simulink model "sampleModel1432_1_sub_sub"  (R2023a)
settings: Solver=VariableStepAuto  StartTime=0.0  StopTime=10.0  RelTol=1e-3
libraries: hdlsllib x5, simulink x2
settings Model: Creator=user1  LastModifiedBy=user1
settings OptimizationCC: BlockReduction=off  ConditionallyExecuteInputs=off

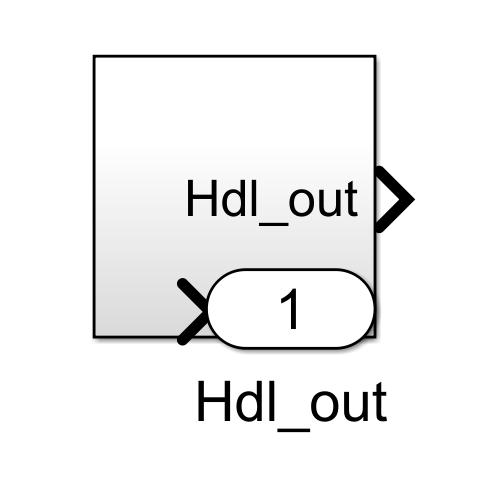
[thumbnail: Simulink's stored preview of the top-level diagram]
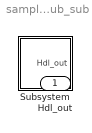
== system sampleModel1432_1_sub_sub ==
  Subsystem : Subsystem
  Hdl_out : Outport  OutDataTypeStr=uint8

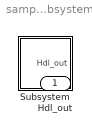
== system sampleModel1432_1_sub_sub/Subsystem ==
  Subsystem : Subsystem
  Hdl_out : Outport  OutDataTypeStr=uint8

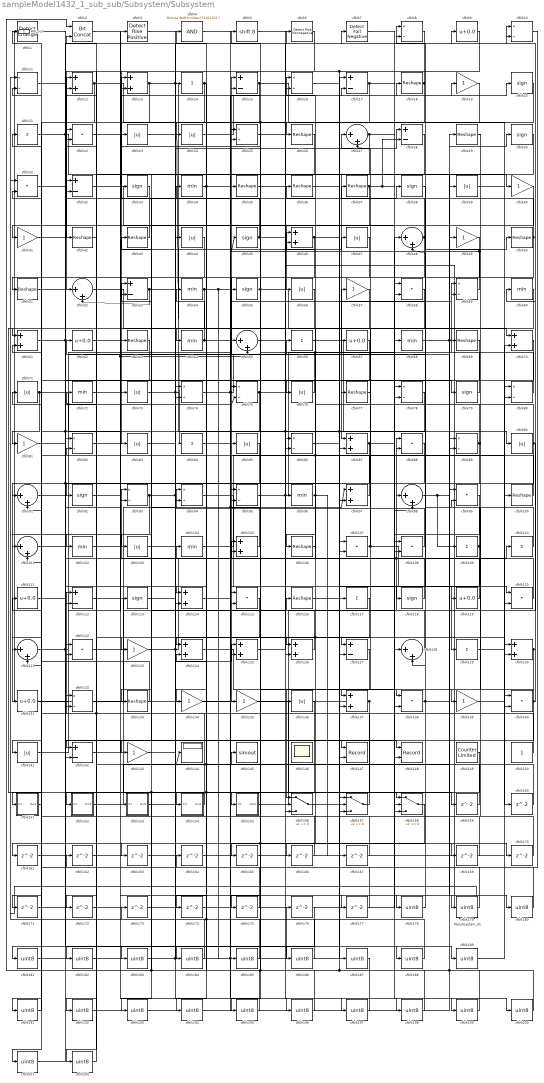
== system sampleModel1432_1_sub_sub/Subsystem/Subsystem ==
  Mysubsystem_31 : Subsystem  TreatAsAtomicUnit=on  RTWFcnName=Mysubsystem_31
      settings: RTWFcnNameOpts=User specified  RTWFileNameOpts=Use function name
  cfblk1 : simulink/Logic and Bit Operations/Detect Change  vinit=0  OutDataTypeStr=uint8
      settings: LibrarySourceBlock=|
      | hdlsllib/Logic and Bit
      | Operations/Detect
      | Change
  cfblk{8,10..11,16,25,59,74..75,78,80,82,86,89,93..95,132} (17 alike) : Product  Inputs=*/  OutDataTypeStr=uint8  RndMeth=Zero  SaturateOnIntegerOverflow=on
  cfblk{18,26,29,35..37,42..43,50..51,63,69,77,100,106,116,133} (17 alike) : Reshape
  cfblk{27,48,52,65,91,98,101,121,128} (9 alike) : Sum  Inputs=|++  OutDataTypeStr=uint8
  cfblk{34,54,60,64,68,72,96,102,104} (9 alike) : MinMax  OutDataTypeStr=uint8
  cfblk{23..24,39,44,47,56,71,73,76,83,85,90,103,136,141} (15 alike) : Abs  OutDataTypeStr=uint8  SaturateOnIntegerOverflow=off
  cfblk{12..13,46,61,70,87,97,105,114,124..126,130,137} (14 alike) : Sum  OutDataTypeStr=uint8
  cfblk{22,31,58,88,99,107..108,115,120,122,138,140} (12 alike) : DotProduct  OutDataTypeStr=uint8
  cfblk{14,21,66,84,109..110,117,129} (8 alike) : Sum  Inputs=+  OutDataTypeStr=uint8
  cfblk{9,62,67,111,119,131} (6 alike) : Bias  Bias=0.0  SaturateOnIntegerOverflow=off
  cfblk{15,17,28,32,53,112,127,142} (8 alike) : Sum  Inputs=+-  OutDataTypeStr=uint8
  cfblk{20,30,33,38,45,55,79,92,113,118} (10 alike) : Signum
  cfblk{19,40..41,49,57,81,123,134..135,139,143} (11 alike) : Gain  OutDataTypeStr=uint8
  cfblk144 : Display
  cfblk145 : ToWorkspace  VariableName=simout  SaveFormat=Timeseries  SampleTime=-1
  cfblk146 : Scope
      settings: Floating=on
  cfblk147 : Record  FileSettingsInternal="{\"entries\":[{\"content\":{\"excelSettings\":{\"content\":{},\"type\":\"Streamout.ExcelSettings\"}},\"type\":\"Streamout.FileSettingStorage\",\"uuid\":\"\"}],\"packageUris\":[\"http:\\/\\/schema.mathworks.com\\/mf0\\/streamout_blocks\\/R2020a\"],\"version\":\"1.0\"}"  Layout=[1 1]  SignalsInternal="{\"entries\":[{\"content\":{\"signals\":[{\"content\":{\"blockPath\":[],\"dimensions\":[1],\"domain\":\"\",\"lineColor\":\"#a2142f\",\"plots\":[1],\"port\":1,\"signalID\":15313,\"signalName\":\"cfblk142\"},\"type\":\"RecordBlkView.Signal\",\"uuid\":\"\"},{\"content\":{\"blockPath\":[],\"dimensions\":[1],\"domain\":\"\",\"lineColor\":\"#139fff\",\"plots\":[1],\"port\":2,\"signalID\":15316,\"signalName\":\"cfblk35\"},\"type\":\"RecordBlkView.Signal\",\"uuid\":\"\"}]},\"type\":\"RecordBlkView.InputSignals\",\"uuid\":\"\"}],\"packageUris\":[\"http:\\/\\/schema.mathworks.com\\/mf0\\/streamout_blocks\\/R2020a\"],\"version\":\"1.0\"}"  VisualizationBindings="{\"xyplotplugin\":{\"info\":[{\"series\":[{\"bindingParametersList\":[{\"parameter\":\"X-Axis\",\"signalID\":15313,\"signalName\":\"cfblk142\"},{\"parameter\":\"Y-Axis\",\"signalID\":15316,\"signalName\":\"cfblk35\"}],\"seriesID\":8691}],\"subplotID\":1}]}}"  CompatibilityTag=XY  st=-1
  cfblk148 : Record  FileSettingsInternal="{\"entries\":[{\"content\":{\"excelSettings\":{\"content\":{},\"type\":\"Streamout.ExcelSettings\"}},\"type\":\"Streamout.FileSettingStorage\",\"uuid\":\"\"}],\"packageUris\":[\"http:\\/\\/schema.mathworks.com\\/mf0\\/streamout_blocks\\/R2020a\"],\"version\":\"1.0\"}"  Layout=[1 1]  SignalsInternal="{\"entries\":[{\"content\":{\"signals\":[{\"content\":{\"blockPath\":[],\"dimensions\":[1],\"domain\":\"\",\"lineColor\":\"#a2142f\",\"plots\":[1],\"port\":1,\"signalID\":15305,\"signalName\":\"cfblk91\"},\"type\":\"RecordBlkView.Signal\",\"uuid\":\"\"},{\"content\":{\"blockPath\":[],\"dimensions\":[1],\"domain\":\"\",\"lineColor\":\"#139fff\",\"plots\":[1],\"port\":2,\"signalID\":15308,\"signalName\":\"cfblk124\"},\"type\":\"RecordBlkView.Signal\",\"uuid\":\"\"}]},\"type\":\"RecordBlkView.InputSignals\",\"uuid\":\"\"}],\"packageUris\":[\"http:\\/\\/schema.mathworks.com\\/mf0\\/streamout_blocks\\/R2020a\"],\"version\":\"1.0\"}"  VisualizationBindings="{\"xyplotplugin\":{\"info\":[{\"series\":[{\"bindingParametersList\":[{\"parameter\":\"X-Axis\",\"signalID\":15305,\"signalName\":\"cfblk91\"},{\"parameter\":\"Y-Axis\",\"signalID\":15308,\"signalName\":\"cfblk124\"}],\"seriesID\":16447}],\"subplotID\":1}]}}"  CompatibilityTag=XY  st=-1
  cfblk149 : hdlsllib/Sources/Counter Limited  uplimit=7  tsamp=-1
  cfblk150 : Constant  OutDataTypeStr=uint8  SampleTime=-1
  cfblk151 : Subsystem
      settings: LibrarySourceBlock=|
      | hdlsllib/Ports &
      | Subsystems/Subsystem
  cfblk152 : Subsystem
      settings: LibrarySourceBlock=|
      | hdlsllib/Ports &
      | Subsystems/Subsystem
  cfblk153 : Subsystem
      settings: LibrarySourceBlock=|
      | hdlsllib/Ports &
      | Subsystems/Subsystem
  cfblk154 : Subsystem
      settings: LibrarySourceBlock=|
      | hdlsllib/Ports &
      | Subsystems/Subsystem
  cfblk155 : Subsystem
      settings: LibrarySourceBlock=|
      | hdlsllib/Ports &
      | Subsystems/Subsystem
  cfblk156 : Switch  OutDataTypeStr=uint8  SaturateOnIntegerOverflow=off  InputSameDT=off
  cfblk157 : Switch  OutDataTypeStr=uint8  SaturateOnIntegerOverflow=off  InputSameDT=off
  cfblk158 : Switch  OutDataTypeStr=uint8  SaturateOnIntegerOverflow=off  InputSameDT=off
  cfblk{159..167,169..177} (18 alike) : Delay  SampleTime=1
  cfblk{178..189,191..202} (24 alike) : DataTypeConversion  OutDataTypeStr=uint8  SaturateOnIntegerOverflow=off  RndMeth=Floor
  cfblk2 : hdlsllib/Logic and Bit Operations/Bit Concat  numInputs=2
  cfblk3 : hdlsllib/Logic and Bit Operations/Detect Rise Positive  vinit=0  OutDataTypeStr=uint8
  cfblk4 : simulink/Logic and Bit Operations/Bitwise Operator  logicop=AND  UseBitMask=on  BitMask=bin2dec('11011001')  BitMaskRealWorld=Stored Integer
      settings: LibrarySourceBlock=|
      | hdlsllib/Logic and Bit
      | Operations/Bitwise
      | Operator
  cfblk5 : ArithShift  BitShiftNumber=8
  cfblk6 : hdlsllib/Logic and Bit Operations/Detect Rise Nonnegative  vinit=0  OutDataTypeStr=uint8
  cfblk7 : hdlsllib/Logic and Bit Operations/Detect Fall Negative  vinit=0  OutDataTypeStr=uint8
  Hdl_out : Outport  OutDataTypeStr=uint8
  wires:
  Mysubsystem_31/1(Out1) -> cfblk11/1
  cfblk202/1 -> cfblk82/2
  cfblk201/1 -> cfblk82/1
  cfblk200/1 -> cfblk122/1, cfblk33/1, cfblk157/2, cfblk89/1
  cfblk199/1 -> cfblk25/2
  cfblk198/1 -> cfblk25/1
  cfblk197/1 -> cfblk173/1, cfblk145/1
  cfblk196/1 -> cfblk35/1
  cfblk4/1 -> cfblk196/1
  cfblk195/1 -> cfblk4/1
  cfblk194/1 -> cfblk115/2
  cfblk193/1 -> cfblk115/1
  cfblk192/1 -> cfblk39/1
  cfblk115/1 -> cfblk192/1
  cfblk191/1 -> cfblk11/2
  cfblk189/1 -> cfblk140/1
  cfblk11/1 -> cfblk189/1
  cfblk188/1 -> cfblk2/2
  cfblk187/1 -> cfblk2/1
  cfblk156/1 -> cfblk187/1
  cfblk186/1 -> cfblk124/2, cfblk144/1, cfblk162/1
  cfblk185/1 -> cfblk31/2
  cfblk184/1 -> cfblk31/1
  cfblk183/1 -> cfblk95/2, cfblk107/1, cfblk74/1
  cfblk182/1 -> cfblk176/1
  cfblk181/1 -> cfblk107/2
  cfblk176/1 -> cfblk181/1
  cfblk180/1 -> cfblk22/2
  cfblk179/1 -> cfblk22/1
  cfblk65/1 -> cfblk179/1
  cfblk178/1 -> cfblk128/2
  cfblk22/1 -> cfblk178/1
  cfblk177/1 -> cfblk132/1
  cfblk3/1 -> cfblk177/1
  cfblk175/1 -> cfblk101/2
  cfblk174/1 -> cfblk128/1
  cfblk20/1 -> cfblk174/1
  cfblk173/1 -> cfblk138/2
  cfblk172/1 -> cfblk105/2
  cfblk171/1 -> cfblk98/2
  cfblk170/1 -> cfblk99/2
  cfblk169/1 -> cfblk1/1
  cfblk114/1 -> cfblk169/1
  cfblk167/1 -> cfblk61/2
  cfblk166/1 -> cfblk53/2
  cfblk165/1 -> cfblk157/1
  cfblk127/1 -> cfblk165/1
  cfblk164/1 -> cfblk70/2
  cfblk10/1 -> cfblk164/1
  cfblk163/1 -> cfblk80/1
  cfblk137/1 -> cfblk163/1, Hdl_out/1
  cfblk162/1 -> cfblk78/2
  cfblk161/1 -> cfblk32/2
  cfblk67/1 -> cfblk161/1
  cfblk160/1 -> cfblk17/1
  cfblk129/1 -> cfblk160/1
  cfblk159/1 -> cfblk12/2
  cfblk87/1 -> cfblk142/2, cfblk120/1
  cfblk32/1 -> cfblk56/1
  cfblk158/1 -> cfblk175/1, cfblk201/1
  cfblk98/1 -> cfblk30/1, cfblk109/1
  cfblk14/1 -> cfblk124/1, cfblk74/2
  cfblk83/1 -> cfblk28/1
  cfblk96/1 -> cfblk166/1, cfblk167/1
  cfblk81/1 -> cfblk97/2, cfblk184/1
  cfblk134/1 -> cfblk17/2, cfblk97/1
  cfblk117/1 -> cfblk136/1, cfblk172/1
  cfblk34/1 -> cfblk114/1, cfblk170/1
  cfblk57/1 -> cfblk106/1
  cfblk152/1(Out1) -> cfblk99/1
  cfblk63/1 -> cfblk142/1
  cfblk80/1 -> cfblk23/1, cfblk46/1
  cfblk139/1 -> cfblk100/1
  cfblk5/1 -> cfblk157/3
  cfblk15/1 -> cfblk130/1, cfblk94/2
  cfblk40/1 -> cfblk123/1
  cfblk66/1 -> cfblk108/2
  cfblk78/1 -> cfblk132/2, cfblk121/2, cfblk156/3
  cfblk82/1 -> cfblk200/1
  cfblk37/1 -> cfblk108/1, cfblk28/2, cfblk61/1
  cfblk8/1 -> cfblk137/2, cfblk156/2
  cfblk108/1 -> cfblk94/1
  cfblk72/1 -> cfblk65/2, cfblk47/1
  cfblk126/1 -> cfblk43/1
  cfblk124/1 -> cfblk148/2
  cfblk35/1 -> cfblk147/2
  cfblk77/1 -> cfblk127/1
  cfblk47/1 -> cfblk141/1
  cfblk38/1 -> cfblk118/1
  cfblk84/1 -> cfblk126/2
  cfblk75/1 -> cfblk58/2, cfblk125/2
  cfblk142/1 -> cfblk147/1
  cfblk122/1 -> cfblk96/1
  cfblk53/1 -> cfblk95/1, cfblk52/2
  cfblk116/1 -> cfblk88/2
  cfblk138/1 -> cfblk49/1, cfblk48/2
  cfblk86/1 -> cfblk59/2
  cfblk52/1 -> cfblk86/1
  cfblk128/1 -> cfblk98/1
  cfblk60/1 -> cfblk137/1
  cfblk111/1 -> cfblk105/1
  cfblk55/1 -> cfblk87/2, cfblk195/1
  cfblk110/1 -> cfblk55/1
  cfblk123/1 -> cfblk58/1, cfblk110/1
  cfblk62/1 -> cfblk113/1
  cfblk151/1(Out1) -> cfblk91/2
  cfblk46/1 -> cfblk152/1(In1), cfblk188/1
  cfblk102/1 -> cfblk3/1
  cfblk68/1 -> cfblk50/1, cfblk180/1
  cfblk104/1 -> cfblk80/2
  cfblk69/1 -> cfblk143/1
  cfblk135/1 -> cfblk158/3
  cfblk36/1 -> cfblk70/1
  cfblk61/1 -> cfblk79/1, cfblk34/1
  cfblk76/1 -> cfblk5/1
  cfblk49/1 -> cfblk85/1
  cfblk140/1 -> cfblk138/1, cfblk10/1, cfblk182/1
  cfblk70/1 -> cfblk133/1
  cfblk125/1 -> cfblk9/1
  cfblk153/1(Out1) -> cfblk125/1
  cfblk56/1 -> cfblk64/1
  cfblk141/1 -> cfblk13/2
  cfblk7/1 -> cfblk68/1
  cfblk29/1 -> cfblk139/1
  cfblk113/1 -> cfblk24/1
  cfblk23/1 -> cfblk78/1
  cfblk85/1 -> cfblk101/1
  cfblk99/1 -> cfblk158/2
  cfblk2/1 -> cfblk186/1
  cfblk27/1 -> cfblk42/1, cfblk199/1
  cfblk30/1 -> cfblk73/1
  cfblk103/1 -> cfblk6/1
  cfblk106/1 -> cfblk126/1
  cfblk44/1 -> cfblk91/1
  cfblk39/1 -> cfblk140/2
  cfblk17/1 -> cfblk40/1, cfblk191/1
  cfblk21/1 -> cfblk69/1, cfblk114/2
  cfblk101/1 -> cfblk93/2
  cfblk16/1 -> cfblk89/2, cfblk159/1
  cfblk45/1 -> Mysubsystem_31/1(In1), cfblk13/1
  cfblk107/1 -> cfblk119/1, cfblk27/2
  cfblk94/1 -> cfblk129/1
  cfblk136/1 -> cfblk155/1(In1)
  cfblk92/1 -> cfblk18/1
  cfblk31/1 -> cfblk183/1
  cfblk12/1 -> cfblk26/1, cfblk51/1
  cfblk105/1 -> cfblk53/1
  cfblk6/1 -> cfblk63/1
  cfblk97/1 -> cfblk15/2
  cfblk9/1 -> cfblk102/1
  cfblk64/1 -> cfblk54/1, cfblk76/1
  cfblk74/1 -> cfblk29/1, cfblk19/1
  cfblk71/1 -> cfblk75/2, cfblk153/1(In1), cfblk81/1
  cfblk143/1 -> cfblk44/1
  cfblk59/1 -> cfblk45/1, cfblk8/1
  cfblk79/1 -> cfblk59/1
  cfblk130/1 -> cfblk156/1, cfblk60/1
  cfblk91/1 -> cfblk148/1
  cfblk1/1 -> cfblk32/1
  cfblk157/1 -> cfblk65/1
  cfblk133/1 -> cfblk111/1
  cfblk154/1(Out1) -> cfblk71/1, cfblk72/1
  cfblk149/1 -> cfblk193/1, cfblk202/1, cfblk194/1
  cfblk51/1 -> cfblk38/1
  cfblk112/1 -> cfblk154/1(In1)
  cfblk73/1 -> cfblk117/1, cfblk198/1
  cfblk33/1 -> cfblk92/1
  cfblk93/1 -> cfblk130/2, cfblk46/2, cfblk151/1(In1)
  cfblk119/1 -> cfblk104/1
  cfblk155/1(Out1) -> cfblk48/1
  cfblk88/1 -> cfblk103/1
  cfblk132/1 -> cfblk14/1
  cfblk100/1 -> cfblk36/1, cfblk21/1
  cfblk24/1 -> cfblk20/1
  cfblk58/1 -> cfblk83/1
  cfblk54/1 -> cfblk120/2, cfblk185/1, cfblk112/2
  cfblk26/1 -> cfblk134/1
  cfblk42/1 -> cfblk158/1
  cfblk19/1 -> cfblk84/1, cfblk75/1
  cfblk50/1 -> cfblk135/1, cfblk27/1
  cfblk95/1 -> cfblk57/1, cfblk7/1
  cfblk43/1 -> cfblk41/1
  cfblk48/1 -> cfblk37/1, cfblk8/2, cfblk171/1
  cfblk41/1 -> cfblk12/1
  cfblk150/1 -> cfblk112/1
  cfblk121/1 -> cfblk15/1, cfblk10/2
  cfblk90/1 -> cfblk116/1, cfblk16/1, cfblk121/1
  cfblk120/1 -> cfblk88/1, cfblk16/2
  cfblk109/1 -> cfblk62/1, cfblk127/2
  cfblk25/1 -> cfblk197/1
  cfblk131/1 -> cfblk66/1
  cfblk89/1 -> cfblk131/1, cfblk67/1
  cfblk18/1 -> cfblk52/1, cfblk86/2
  cfblk118/1 -> cfblk93/1
  cfblk28/1 -> cfblk87/1
  cfblk13/1 -> cfblk90/1, cfblk77/1, cfblk122/2

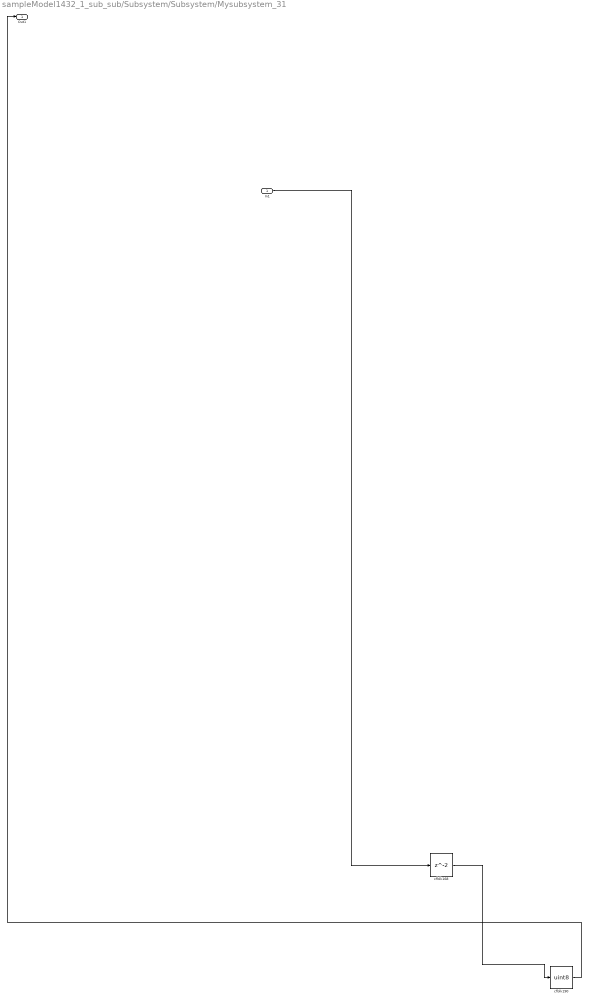
== system sampleModel1432_1_sub_sub/Subsystem/Subsystem/Mysubsystem_31 ==
  In1 : Inport
  cfblk168 : Delay  SampleTime=1
  cfblk190 : DataTypeConversion  OutDataTypeStr=uint8  SaturateOnIntegerOverflow=off  RndMeth=Floor
  Out1 : Outport
  wires:
  cfblk168/1 -> cfblk190/1
  cfblk190/1 -> Out1/1
  In1/1 -> cfblk168/1

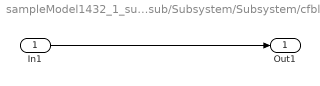
== system sampleModel1432_1_sub_sub/Subsystem/Subsystem/cfblk151 ==
  In1 : Inport
  Out1 : Outport
  wires:
  In1/1 -> Out1/1

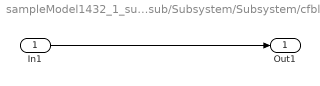
== system sampleModel1432_1_sub_sub/Subsystem/Subsystem/cfblk152 ==
  In1 : Inport
  Out1 : Outport
  wires:
  In1/1 -> Out1/1

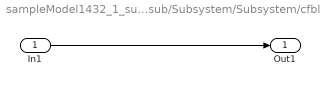
== system sampleModel1432_1_sub_sub/Subsystem/Subsystem/cfblk153 ==
  In1 : Inport
  Out1 : Outport
  wires:
  In1/1 -> Out1/1

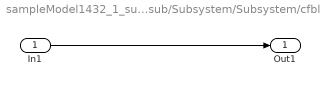
== system sampleModel1432_1_sub_sub/Subsystem/Subsystem/cfblk154 ==
  In1 : Inport
  Out1 : Outport
  wires:
  In1/1 -> Out1/1

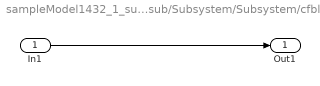
== system sampleModel1432_1_sub_sub/Subsystem/Subsystem/cfblk155 ==
  In1 : Inport
  Out1 : Outport
  wires:
  In1/1 -> Out1/1
